simulink model "TestModel"  (R2016a)
settings: Solver=FixedStepAuto  StartTime=0.0  StopTime=10.0  RelTol=1e-3
undefined symbols (not defined in the file): f1, f2, tau
settings Model: Creator=ich  LastModifiedBy=ich

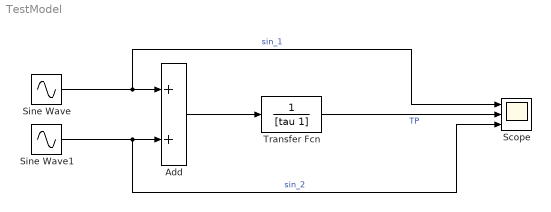
== system TestModel ==
  Add : Sum
  Scope : Scope  NumInputPorts=3
  Sine Wave : Sin  Frequency=2*pi*f1
  Sine Wave1 : Sin  Frequency=2*pi*f2
  Transfer Fcn : TransferFcn  Denominator=[tau 1]
  wires:
  Sine Wave/1 -> Scope/1, Add/1  "sin_1"
  Sine Wave1/1 -> Scope/3, Add/2  "sin_2"
  Add/1 -> Transfer Fcn/1
  Transfer Fcn/1 -> Scope/2  "TP"
